simulink model "ES106A_StHlthSigStc"  (R2013b)
settings: Solver=FixedStepDiscrete  SolverMode=SingleTasking  StartTime=0.0  StopTime=1  FixedStep=0.002  RelTol=1e-3
undefined symbols (not defined in the file): APPL10_CNT_U08, BITSPERBYTE_CNT_U08, ENOTOK_CNT_U08, EOK_CNT_U08, LOWRMASKVAL_CNT_U32, NROFCRCAREA_CNT_U08, NVMAVRGPOSN_CNT_U08, NvmGetErrSts1, NVMMAXPOSN_CNT_U08, NVMMINPOSN_CNT_U08, NVMSAMPLECNTRPOSN_CNT_U08, RAMMAXPOSN_CNT_U08, RAMMINPOSN_CNT_U08, RAMRAWPOSN_CNT_U08, SIGCNT_ULS_U08, SigStcPrmInst, STHLTHMAXVAL_CNT_U08, STHLTHOSAPPL_CNT_U16, StHlthTaskRef1, WORDSIZE_CNT_U08
libraries: simulink x43, NxtrNvM x4, NxtrMax x4, NxtrMin x4, FloatToFixd x3, NxtrLim x2
(part 4 of 5)

== system ES106A_StHlthSigStc/StHlthSigStc/GetSigStcHlthData/If Action Subsystem1/GetSigStcHlthData/Subsystem1 ==
  In1 : Inport
  Bitwise Operator1 : simulink/Logic and Bit Operations/Bitwise Operator  logicop=AND  UseBitMask=on  BitMask=bin2dec('1111111100000000')  BitMaskRealWorld=Stored Integer
  Bitwise Operator2 : simulink/Logic and Bit Operations/Bitwise Operator  logicop=AND  UseBitMask=on  BitMask=bin2dec('11111111')  BitMaskRealWorld=Stored Integer
  CopyRight2 : Subsystem  Description=|  mask(Copyright Information){none=on}
      | Copyright info block.                                               
      |                                                                     
      | Place copyright information at the top of every subsystem in design.
      mask prompts: none "No parameters"
      mask help: Place copyright information at the top of every subsystem in design.
      mask Display:
      | NxtrConf = 'Nexteer Confidential';
      | 
      | sys = bdroot; %handle for the current model ("system")
      | first = get_param(sys,'Created');
      | first = first(end-3:end);  %year is last four digits
      | 
      | last = get_param(sys,'LastModifiedDate');
      | if isempty(last)
      |     last = datestr(now,'yyyy');
      | else
      |     last = last(end-3:end);
      | end
      | 
      | if strcmp(first,last)
      |     fprintf('%s -- Copyright %s Nexteer',NxtrConf,first)
      | else
      |     fprintf('%s -- %s%s- %s Nexteer',NxtrConf,char(169),first,last)
      | end
  Data Type Conversion2 : DataTypeConversion  OutDataTypeStr=uint8
  Data Type Conversion3 : DataTypeConversion  OutDataTypeStr=uint8
  Shift Arithmetic2 : ArithShift  BitShiftNumber=8  BitShiftDirection=Right
  Out1 : Outport
  Out2 : Outport  Port=2
  wires:
  Shift Arithmetic2/1 -> Data Type Conversion2/1
  In1/1 -> Bitwise Operator2/1, Bitwise Operator1/1
  Bitwise Operator2/1 -> Data Type Conversion3/1
  Bitwise Operator1/1 -> Shift Arithmetic2/1
  Data Type Conversion2/1 -> Out1/1
  Data Type Conversion3/1 -> Out2/1

== system ES106A_StHlthSigStc/StHlthSigStc/GetSigStcHlthData/If Action Subsystem1/GetSigStcHlthData/Subsystem2 ==
  In1 : Inport
  Bitwise Operator1 : simulink/Logic and Bit Operations/Bitwise Operator  logicop=AND  UseBitMask=on  BitMask=bin2dec('1111111100000000')  BitMaskRealWorld=Stored Integer
  Bitwise Operator2 : simulink/Logic and Bit Operations/Bitwise Operator  logicop=AND  UseBitMask=on  BitMask=bin2dec('11111111')  BitMaskRealWorld=Stored Integer
  CopyRight2 : Subsystem  Description=|  mask(Copyright Information){none=on}
      | Copyright info block.                                               
      |                                                                     
      | Place copyright information at the top of every subsystem in design.
      mask prompts: none "No parameters"
      mask help: Place copyright information at the top of every subsystem in design.
      mask Display:
      | NxtrConf = 'Nexteer Confidential';
      | 
      | sys = bdroot; %handle for the current model ("system")
      | first = get_param(sys,'Created');
      | first = first(end-3:end);  %year is last four digits
      | 
      | last = get_param(sys,'LastModifiedDate');
      | if isempty(last)
      |     last = datestr(now,'yyyy');
      | else
      |     last = last(end-3:end);
      | end
      | 
      | if strcmp(first,last)
      |     fprintf('%s -- Copyright %s Nexteer',NxtrConf,first)
      | else
      |     fprintf('%s -- %s%s- %s Nexteer',NxtrConf,char(169),first,last)
      | end
  Data Type Conversion2 : DataTypeConversion  OutDataTypeStr=uint8
  Data Type Conversion3 : DataTypeConversion  OutDataTypeStr=uint8
  Shift Arithmetic2 : ArithShift  BitShiftNumber=8  BitShiftDirection=Right
  Out1 : Outport
  Out2 : Outport  Port=2
  wires:
  Shift Arithmetic2/1 -> Data Type Conversion2/1
  In1/1 -> Bitwise Operator2/1, Bitwise Operator1/1
  Bitwise Operator2/1 -> Data Type Conversion3/1
  Bitwise Operator1/1 -> Shift Arithmetic2/1
  Data Type Conversion2/1 -> Out1/1
  Data Type Conversion3/1 -> Out2/1

== system ES106A_StHlthSigStc/StHlthSigStc/GetSigStcHlthData/If Action Subsystem1/GetSigStcHlthData/SuspendAllInterrupts ==

== system ES106A_StHlthSigStc/StHlthSigStc/GetSigStcHlthData/If Action Subsystem1/If Action Subsystem/CopyRight2 ==

== system ES106A_StHlthSigStc/StHlthSigStc/StHlthSigStcInit1/Check Applicability/Do Nothing/Subsystem5 ==

== system ES106A_StHlthSigStc/StHlthSigStc/StHlthSigStcInit1/Check Applicability/Set Nvm Invalid/Subsystem5 ==

== system ES106A_StHlthSigStc/StHlthSigStc/StHlthSigStcInit1/For Simulation Purpose/Merger/CopyRight2 ==

== system ES106A_StHlthSigStc/StHlthSigStc/StHlthSigStcInit1/Prepare a buffer for CRC calculation/Iterator/CopyRight2 ==

== system ES106A_StHlthSigStc/StHlthSigStc/StHlthStcPwrDwn/For Iterator Subsystem/If Action Subsystem/ Ignition cycle lasts for less than 1 second. ==
  RamMaxVal : Inport
  RamMinVal : Inport  Port=2
  SigAvrgVal : Inport  Port=3
  SampleCnt : Inport  Port=4
  Action Port : ActionPort  ActionType=else
  CopyRight2 : Subsystem  Description=|  mask(Copyright Information){none=on}
      | Copyright info block.                                               
      |                                                                     
      | Place copyright information at the top of every subsystem in design.
      mask prompts: none "No parameters"
      mask help: Place copyright information at the top of every subsystem in design.
      mask Display:
      | NxtrConf = 'Nexteer Confidential';
      | 
      | sys = bdroot; %handle for the current model ("system")
      | first = get_param(sys,'Created');
      | first = first(end-3:end);  %year is last four digits
      | 
      | last = get_param(sys,'LastModifiedDate');
      | if isempty(last)
      |     last = datestr(now,'yyyy');
      | else
      |     last = last(end-3:end);
      | end
      | 
      | if strcmp(first,last)
      |     fprintf('%s -- Copyright %s Nexteer',NxtrConf,first)
      | else
      |     fprintf('%s -- %s%s- %s Nexteer',NxtrConf,char(169),first,last)
      | end
  NvmMaxVal : Outport
  NvmMinVal : Outport  Port=2
  NvmAvrgVal : Outport  Port=3
  NvmSampleCnt : Outport  Port=4
  wires:
  RamMaxVal/1 -> NvmMaxVal/1
  RamMinVal/1 -> NvmMinVal/1
  SampleCnt/1 -> NvmSampleCnt/1
  SigAvrgVal/1 -> NvmAvrgVal/1

== system ES106A_StHlthSigStc/StHlthSigStc/StHlthStcPwrDwn/For Iterator Subsystem/If Action Subsystem/CopyRight2 ==

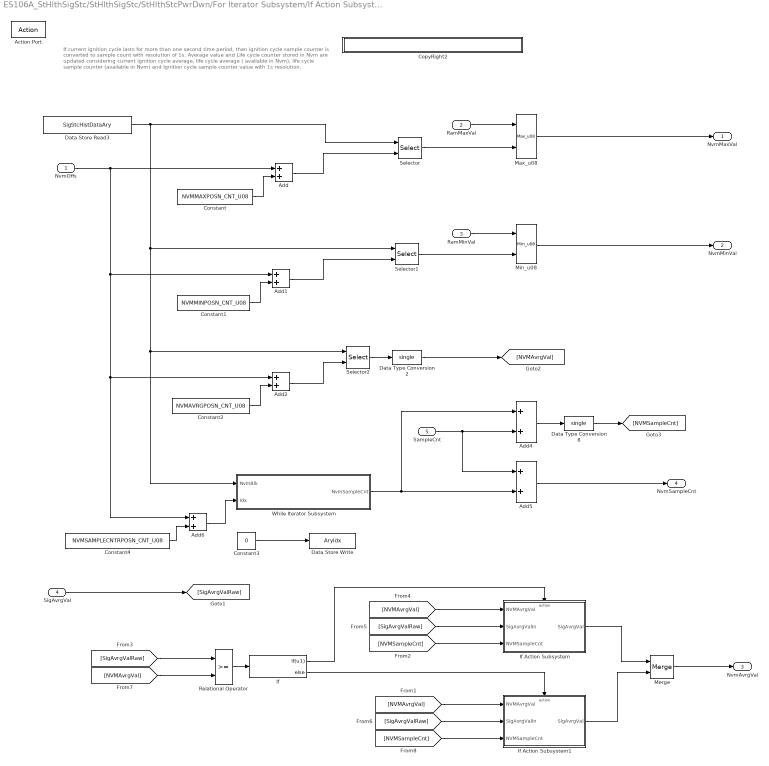
== system ES106A_StHlthSigStc/StHlthSigStc/StHlthStcPwrDwn/For Iterator Subsystem/If Action Subsystem/Statistical data computation for Controller Life Cycle ==
  note: If current ignition cycle lasts for more than one second time period, then ignition cycle sample counter
      | is converted to sample count with resolution of 1s. Average value and Life cycle counter stored in Nvm
      | are updated considering current ignition cycle average, life cycle average ( available in Nvm),
      | life cycle sample counter (available in Nvm) and Ignition cycle sample counter value with 1s resolution.
  NvmOffs : Inport
  RamMaxVal : Inport  Port=2
  RamMinVal : Inport  Port=3
  SigAvrgVal : Inport  Port=4
  SampleCnt : Inport  Port=5
  Action Port : ActionPort  ActionType=then
  Add{,1..2,4..6} (6 alike) : Sum
  Constant : Constant  Value=NVMMAXPOSN_CNT_U08  OutDataTypeStr=uint8
  Constant1 : Constant  Value=NVMMINPOSN_CNT_U08  OutDataTypeStr=uint8
  Constant2 : Constant  Value=NVMAVRGPOSN_CNT_U08  OutDataTypeStr=uint8
  Constant3 : Constant  Value=0
  Constant4 : Constant  Value=NVMSAMPLECNTRPOSN_CNT_U08  OutDataTypeStr=uint8
  CopyRight2 : Subsystem  Description=|  mask(Copyright Information){none=on}
      | Copyright info block.                                               
      |                                                                     
      | Place copyright information at the top of every subsystem in design.
      mask prompts: none "No parameters"
      mask help: Place copyright information at the top of every subsystem in design.
      mask Display:
      | NxtrConf = 'Nexteer Confidential';
      | 
      | sys = bdroot; %handle for the current model ("system")
      | first = get_param(sys,'Created');
      | first = first(end-3:end);  %year is last four digits
      | 
      | last = get_param(sys,'LastModifiedDate');
      | if isempty(last)
      |     last = datestr(now,'yyyy');
      | else
      |     last = last(end-3:end);
      | end
      | 
      | if strcmp(first,last)
      |     fprintf('%s -- Copyright %s Nexteer',NxtrConf,first)
      | else
      |     fprintf('%s -- %s%s- %s Nexteer',NxtrConf,char(169),first,last)
      | end
  Data Store Read3 : DataStoreRead  DataStoreName=SigStcHistDataAry
  Data Store Write : DataStoreWrite  Priority=2  DataStoreName=AryIdx
  Data Type Conversion2 : DataTypeConversion  OutDataTypeStr=single
  Data Type Conversion8 : DataTypeConversion  OutDataTypeStr=single
  If : If  IfExpression=u1
  If Action Subsystem : Subsystem  TreatAsAtomicUnit=on
  If Action Subsystem1 : Subsystem  TreatAsAtomicUnit=on
  Max_u08 : NxtrMax/Max_u08  SFunctionSpec="uint8 y1 = Max_u08( uint8 u1,  uint8 u2)"
      settings: AttributesFormatString=%<Name>
  Merge : Merge
  Min_u08 : NxtrMin/Min_u08  SFunctionSpec="uint8 y1 = Min_u08( uint8 u1,  uint8 u2)"  ShowSpec=off
      settings: AttributesFormatString=%<Name>
  Relational Operator : RelationalOperator  OutDataTypeStr=boolean
  Selector : Selector  IndexMode=Zero-based  InputPortWidth=225  IndexOptions=Starting index (port)  Indices=[1 3]  OutputSizes=1
  Selector1 : Selector  IndexMode=Zero-based  InputPortWidth=225  IndexOptions=Starting index (port)  Indices=[1 3]  OutputSizes=1
  Selector2 : Selector  IndexMode=Zero-based  InputPortWidth=225  IndexOptions=Starting index (port)  Indices=[1 3]  OutputSizes=1
  While Iterator Subsystem : Subsystem  TreatAsAtomicUnit=on
  NvmMaxVal : Outport
  NvmMinVal : Outport  Port=2
  NvmAvrgVal : Outport  Port=3
  NvmSampleCnt : Outport  Port=4
  wires:
  Constant/1 -> Add/2
  Add/1 -> Selector/2
  Constant1/1 -> Add1/2
  Add1/1 -> Selector1/2
  NvmOffs/1 -> Add6/1, Add2/1, Add1/1, Add/1
  Constant2/1 -> Add2/2
  Add2/1 -> Selector2/2
  RamMaxVal/1 -> Max_u08/1
  Selector/1 -> Max_u08/2
  Max_u08/1 -> NvmMaxVal/1
  RamMinVal/1 -> Min_u08/1
  Selector1/1 -> Min_u08/2
  Min_u08/1 -> NvmMinVal/1
  Selector2/1 -> Data Type Conversion2/1
  SampleCnt/1 -> Add5/1, Add4/2
  Add4/1 -> Data Type Conversion8/1
  Add5/1 -> NvmSampleCnt/1
  While Iterator Subsystem/1(NvmSampleCnt) -> Add5/2, Add4/1
  Add6/1 -> While Iterator Subsystem/2(Idx)
  Constant4/1 -> Add6/2
  Constant3/1 -> Data Store Write/1
  Data Store Read3/1 -> Selector2/1, While Iterator Subsystem/1(NvmBlk), Selector1/1, Selector/1
  Relational Operator/1 -> If/1
  If/1 -> If Action Subsystem/Action
  If/2 -> If Action Subsystem1/Action
  Merge/1 -> NvmAvrgVal/1
  If Action Subsystem/1(SigAvrgVal) -> Merge/1
  If Action Subsystem1/1(SigAvrgVal) -> Merge/2
  [NVMAvrgVal] -> If Action Subsystem/1(NVMAvrgVal)
  [NVMAvrgVal] -> If Action Subsystem1/1(NVMAvrgVal)
  [SigAvrgValRaw] -> Relational Operator/1
  Data Type Conversion2/1 -> [NVMAvrgVal]
  [NVMAvrgVal] -> Relational Operator/2
  [NVMSampleCnt] -> If Action Subsystem1/3(NVMSampleCnt)
  [SigAvrgValRaw] -> If Action Subsystem/2(SigAvrgValIn)
  [NVMSampleCnt] -> If Action Subsystem/3(NVMSampleCnt)
  [SigAvrgValRaw] -> If Action Subsystem1/2(SigAvrgValIn)
  SigAvrgVal/1 -> [SigAvrgValRaw]
  Data Type Conversion8/1 -> [NVMSampleCnt]

== system ES106A_StHlthSigStc/StHlthSigStc/StHlthStcPwrDwn/For Iterator Subsystem/If Action Subsystem/Update Nvm ==
  NvmOffset : Inport
  MaxVal : Inport  Port=2
  MinVal : Inport  Port=3
  AvgVal : Inport  Port=4
  SampleCnt : Inport  Port=5
  Assignment : Assignment  IndexMode=Zero-based  IndexOptions=Starting index (port)  Indices=1  OutputSizes=1
  CopyRight2 : Subsystem  Description=|  mask(Copyright Information){none=on}
      | Copyright info block.                                               
      |                                                                     
      | Place copyright information at the top of every subsystem in design.
      mask prompts: none "No parameters"
      mask help: Place copyright information at the top of every subsystem in design.
      mask Display:
      | NxtrConf = 'Nexteer Confidential';
      | 
      | sys = bdroot; %handle for the current model ("system")
      | first = get_param(sys,'Created');
      | first = first(end-3:end);  %year is last four digits
      | 
      | last = get_param(sys,'LastModifiedDate');
      | if isempty(last)
      |     last = datestr(now,'yyyy');
      | else
      |     last = last(end-3:end);
      | end
      | 
      | if strcmp(first,last)
      |     fprintf('%s -- Copyright %s Nexteer',NxtrConf,first)
      | else
      |     fprintf('%s -- %s%s- %s Nexteer',NxtrConf,char(169),first,last)
      | end
  Data Store Read7 : DataStoreRead  DataStoreName=SigStcHistDataAry
  Data Store Write1 : DataStoreWrite  DataStoreName=SigStcHistDataAry
  FloatToFixd_u16_f32 : FloatToFixd/FloatToFixd_u16_f32  Param1=9
  Mux : Mux  Inputs=8
  Subsystem : Subsystem
  Subsystem1 : Subsystem
  wires:
  SampleCnt/1 -> Subsystem/1(In1)
  Assignment/1 -> Data Store Write1/1
  Data Store Read7/1 -> Assignment/1
  Mux/1 -> Assignment/2
  NvmOffset/1 -> Assignment/3
  MaxVal/1 -> Mux/1
  MinVal/1 -> Mux/2
  Subsystem/1(Out1) -> Mux/5
  Subsystem/2(Out2) -> Mux/6
  Subsystem/3(Out3) -> Mux/7
  Subsystem/4(Out4) -> Mux/8
  AvgVal/1 -> FloatToFixd_u16_f32/1
  Subsystem1/1(Out1) -> Mux/3
  Subsystem1/2(Out2) -> Mux/4
  FloatToFixd_u16_f32/1 -> Subsystem1/1(In1)

== system ES106A_StHlthSigStc/StHlthSigStc/UpdStHlthStcData/Call Non Trusted Function /For Iterator Subsystem/CopyRight2 ==

== system ES106A_StHlthSigStc/StHlthSigStc/UpdStHlthStcData/Call Non Trusted Function /For Iterator Subsystem/If Action Subsystem2 ==
  note: /*Do Nothing*/
  Action Port : ActionPort  ActionType=else
  CopyRight2 : Subsystem  Description=|  mask(Copyright Information){none=on}
      | Copyright info block.                                               
      |                                                                     
      | Place copyright information at the top of every subsystem in design.
      mask prompts: none "No parameters"
      mask help: Place copyright information at the top of every subsystem in design.
      mask Display:
      | NxtrConf = 'Nexteer Confidential';
      | 
      | sys = bdroot; %handle for the current model ("system")
      | first = get_param(sys,'Created');
      | first = first(end-3:end);  %year is last four digits
      | 
      | last = get_param(sys,'LastModifiedDate');
      | if isempty(last)
      |     last = datestr(now,'yyyy');
      | else
      |     last = last(end-3:end);
      | end
      | 
      | if strcmp(first,last)
      |     fprintf('%s -- Copyright %s Nexteer',NxtrConf,first)
      | else
      |     fprintf('%s -- %s%s- %s Nexteer',NxtrConf,char(169),first,last)
      | end

== system ES106A_StHlthSigStc/StHlthSigStc/UpdStHlthStcData/Call Non Trusted Function /For Iterator Subsystem/Subsystem2 ==
  note: The Function pointer is terminated in the model to indicate that the pointer
      | points to a location that is outside this FDD. And whiile coding, this pointer is used
      | to access information that is generated from other components.
  FunPtr : Inport
  RAMOffset : Inport  Port=2
  SigIdx : Inport  Port=3
  StHlthSig : Inport  Port=4
  Action Port : ActionPort  ActionType=then
  CopyRight2 : Subsystem  Description=|  mask(Copyright Information){none=on}
      | Copyright info block.                                               
      |                                                                     
      | Place copyright information at the top of every subsystem in design.
      mask prompts: none "No parameters"
      mask help: Place copyright information at the top of every subsystem in design.
      mask Display:
      | NxtrConf = 'Nexteer Confidential';
      | 
      | sys = bdroot; %handle for the current model ("system")
      | first = get_param(sys,'Created');
      | first = first(end-3:end);  %year is last four digits
      | 
      | last = get_param(sys,'LastModifiedDate');
      | if isempty(last)
      |     last = datestr(now,'yyyy');
      | else
      |     last = last(end-3:end);
      | end
      | 
      | if strcmp(first,last)
      |     fprintf('%s -- Copyright %s Nexteer',NxtrConf,first)
      | else
      |     fprintf('%s -- %s%s- %s Nexteer',NxtrConf,char(169),first,last)
      | end
  If Action Subsystem : Subsystem  RequirementInfo={'linktype_rmi_doors' '0001022b (/ESG Group/FDD Module Requirements/EA4 Specific/ES106A_StHlthSigStc )' '#ES106A_15' 'true' 'REQ:ES106A_15' '' ; 'linktype_rmi_doors' '0001022b (/ESG Group/FDD Module Requirements/EA4 Specific/ES106A_StHlthSigStc )' '#ES106A_18' 'true' 'REQ:ES106A_18' '' ; 'linktype_rmi_doors' '0001022b (/ESG Group/FDD Module Requirements/EA4 Specific/ES106A_StHlthSigStc )' '#ES106A_21' 'true' 'REQ:ES106A_21' '' ; 'linktype_rmi_doors' '0001022b (/ESG Group/FDD Module Requirements/EA4 Specific/ES106A_StHlthSigStc )' '#ES106A_22' 'true' 'REQ:ES106A_22' '' } %GIDa_4259b254_6da3_458f_aa6d_9446d195bc64  TreatAsAtomicUnit=on
  Selector : Selector  IndexMode=Zero-based  InputPortWidth=22  IndexOptions=Starting index (port)  Indices=[1 3]  OutputSizes=1
  Terminator : Terminator
  UpdateRamBuf : Subsystem
  UpdateSigAvrgBuf : Subsystem
  wires:
  FunPtr/1 -> Terminator/1
  StHlthSig/1 -> Selector/1
  SigIdx/1 -> [SigIdxVal], Selector/2
  [SigIdxVal] -> If Action Subsystem/1(SigIdx)
  Selector/1 -> If Action Subsystem/2(StHlthSig)
  RAMOffset/1 -> [RAMOffset], If Action Subsystem/3(RAMOffset)
  [RAMOffset] -> UpdateRamBuf/1(RAMLocation)
  If Action Subsystem/1(RamRawVal) -> UpdateRamBuf/2(RamRawVal)
  If Action Subsystem/2(RamMaxVal) -> UpdateRamBuf/3(RamMaxVal)
  If Action Subsystem/3(RamMinVal) -> UpdateRamBuf/4(RamMinVal)
  [SigIdxVal] -> [SigOffset], If Action Subsystem/4(SigOffset)
  [SigOffset] -> UpdateSigAvrgBuf/1(SigAvrgLocation)
  If Action Subsystem/4(SigAvrgVal) -> UpdateSigAvrgBuf/2(SigAvrgVal)

== system ES106A_StHlthSigStc/StHlthSigStc/UpdStHlthStcData/UpdDataSample/For Iterator Subsystem/CopyRight2 ==

== system ES106A_StHlthSigStc/StHlthSigStc/UpdStHlthStcData/UpdDataSample/For Iterator Subsystem/If Action Subsystem2 ==
  note: /*Do Nothing*/
  Action Port : ActionPort  ActionType=else
  CopyRight2 : Subsystem  Description=|  mask(Copyright Information){none=on}
      | Copyright info block.                                               
      |                                                                     
      | Place copyright information at the top of every subsystem in design.
      mask prompts: none "No parameters"
      mask help: Place copyright information at the top of every subsystem in design.
      mask Display:
      | NxtrConf = 'Nexteer Confidential';
      | 
      | sys = bdroot; %handle for the current model ("system")
      | first = get_param(sys,'Created');
      | first = first(end-3:end);  %year is last four digits
      | 
      | last = get_param(sys,'LastModifiedDate');
      | if isempty(last)
      |     last = datestr(now,'yyyy');
      | else
      |     last = last(end-3:end);
      | end
      | 
      | if strcmp(first,last)
      |     fprintf('%s -- Copyright %s Nexteer',NxtrConf,first)
      | else
      |     fprintf('%s -- %s%s- %s Nexteer',NxtrConf,char(169),first,last)
      | end

== system ES106A_StHlthSigStc/StHlthSigStc/UpdStHlthStcData/UpdDataSample/For Iterator Subsystem/Subsystem2 ==
  note: The Function pointer is terminated in the model to indicate that the pointer
      | points to a location that is outside this FDD. And whiile coding, this pointer is used
      | to access information that is generated from other components.
  FunPtr : Inport
  RAMOffset : Inport  Port=2
  SigIdx : Inport  Port=3
  StHlthSig : Inport  Port=4
  Action Port : ActionPort  ActionType=then
  CopyRight2 : Subsystem  Description=|  mask(Copyright Information){none=on}
      | Copyright info block.                                               
      |                                                                     
      | Place copyright information at the top of every subsystem in design.
      mask prompts: none "No parameters"
      mask help: Place copyright information at the top of every subsystem in design.
      mask Display:
      | NxtrConf = 'Nexteer Confidential';
      | 
      | sys = bdroot; %handle for the current model ("system")
      | first = get_param(sys,'Created');
      | first = first(end-3:end);  %year is last four digits
      | 
      | last = get_param(sys,'LastModifiedDate');
      | if isempty(last)
      |     last = datestr(now,'yyyy');
      | else
      |     last = last(end-3:end);
      | end
      | 
      | if strcmp(first,last)
      |     fprintf('%s -- Copyright %s Nexteer',NxtrConf,first)
      | else
      |     fprintf('%s -- %s%s- %s Nexteer',NxtrConf,char(169),first,last)
      | end
  If Action Subsystem : Subsystem  RequirementInfo={'linktype_rmi_doors' '0001022b (/ESG Group/FDD Module Requirements/EA4 Specific/ES106A_StHlthSigStc )' '#ES106A_15' 'true' 'REQ:ES106A_15' '' ; 'linktype_rmi_doors' '0001022b (/ESG Group/FDD Module Requirements/EA4 Specific/ES106A_StHlthSigStc )' '#ES106A_18' 'true' 'REQ:ES106A_18' '' ; 'linktype_rmi_doors' '0001022b (/ESG Group/FDD Module Requirements/EA4 Specific/ES106A_StHlthSigStc )' '#ES106A_21' 'true' 'REQ:ES106A_21' '' ; 'linktype_rmi_doors' '0001022b (/ESG Group/FDD Module Requirements/EA4 Specific/ES106A_StHlthSigStc )' '#ES106A_22' 'true' 'REQ:ES106A_22' '' } %GIDa_dda2dc3d_9a01_4c14_a4da_d10ab0df32b8  TreatAsAtomicUnit=on
  Selector : Selector  IndexMode=Zero-based  InputPortWidth=22  IndexOptions=Starting index (port)  Indices=[1 3]  OutputSizes=1
  Terminator : Terminator
  UpdateRamBuf : Subsystem
  UpdateSigAvrgBuf : Subsystem
  wires:
  FunPtr/1 -> Terminator/1
  StHlthSig/1 -> Selector/1
  SigIdx/1 -> [SigIdxVal], Selector/2
  [SigIdxVal] -> If Action Subsystem/1(SigIdx)
  Selector/1 -> If Action Subsystem/2(StHlthSig)
  RAMOffset/1 -> [RAMOffset], If Action Subsystem/3(RAMOffset)
  [RAMOffset] -> UpdateRamBuf/1(RAMLocation)
  If Action Subsystem/1(RamRawVal) -> UpdateRamBuf/2(RamRawVal)
  If Action Subsystem/2(RamMaxVal) -> UpdateRamBuf/3(RamMaxVal)
  If Action Subsystem/3(RamMinVal) -> UpdateRamBuf/4(RamMinVal)
  [SigIdxVal] -> [SigOffset], If Action Subsystem/4(SigAvrgOffset)
  [SigOffset] -> UpdateSigAvrgBuf/1(SigAvrgLocation)
  If Action Subsystem/4(SigAvrgVal) -> UpdateSigAvrgBuf/2(SigAvrgVal)

== system ES106A_StHlthSigStc/StHlthSigStc/GetSigStcHlthData/If Action Subsystem1/GetSigStcHlthData/If Action Subsystem/CopyRight2 ==

== system ES106A_StHlthSigStc/StHlthSigStc/GetSigStcHlthData/If Action Subsystem1/GetSigStcHlthData/If Action Subsystem/If Action Subsystem ==
  NVMAvrgVal : Inport
  SigAvrgValIn : Inport  Port=2
  NVMSampleCnt : Inport  Port=3
  Action Port : ActionPort  ActionType=then
  Add1 : Sum
  Add4 : Sum  Inputs=+-
  Divide : Product  Inputs=*/
  SigAvrgVal : Outport
  wires:
  [SigAvrgVal] -> Add4/1
  NVMAvrgVal/1 -> [NVMAvrgVal]
  Add4/1 -> Divide/1
  NVMSampleCnt/1 -> Divide/2
  SigAvrgValIn/1 -> [SigAvrgVal]
  Divide/1 -> Add1/2
  [NVMAvrgVal] -> Add1/1
  Add1/1 -> SigAvrgVal/1
  [NVMAvrgVal] -> Add4/2

== system ES106A_StHlthSigStc/StHlthSigStc/GetSigStcHlthData/If Action Subsystem1/GetSigStcHlthData/If Action Subsystem/If Action Subsystem1 ==
  NVMAvrgVal : Inport
  SigAvrgValIn : Inport  Port=2
  NVMSampleCnt : Inport  Port=3
  Action Port : ActionPort  ActionType=else
  Add1 : Sum  Inputs=+-
  Add4 : Sum  Inputs=+-
  Divide : Product  Inputs=*/
  SigAvrgVal : Outport
  wires:
  [SigAvrgVal] -> Add4/2
  NVMAvrgVal/1 -> [NVMAvrgVal]
  Add4/1 -> Divide/1
  NVMSampleCnt/1 -> Divide/2
  SigAvrgValIn/1 -> [SigAvrgVal]
  Divide/1 -> Add1/2
  [NVMAvrgVal] -> Add1/1
  Add1/1 -> SigAvrgVal/1
  [NVMAvrgVal] -> Add4/1

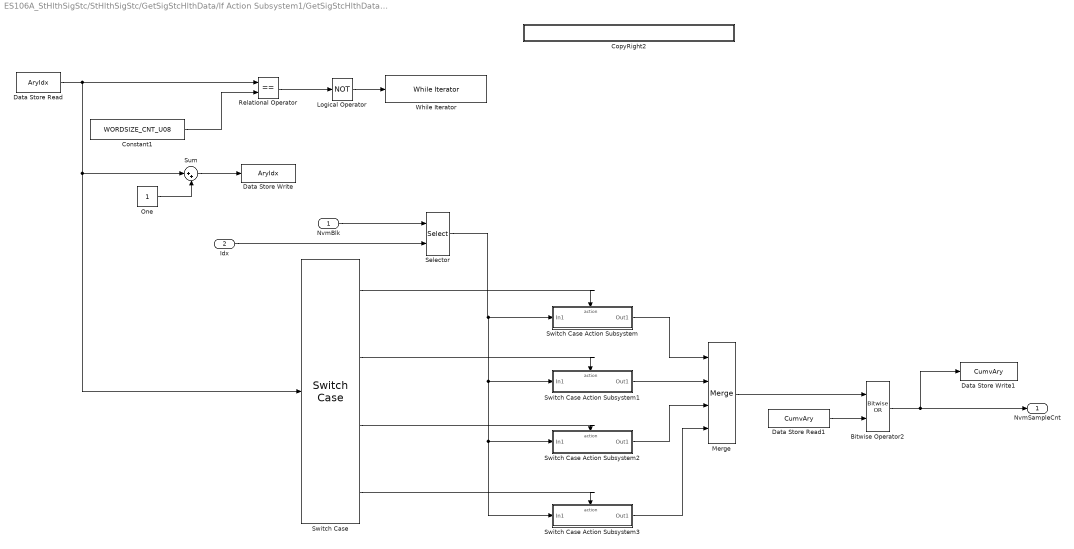
== system ES106A_StHlthSigStc/StHlthSigStc/GetSigStcHlthData/If Action Subsystem1/GetSigStcHlthData/If Action Subsystem/While Iterator Subsystem ==
  NvmBlk : Inport
  Idx : Inport  Port=2
  Bitwise Operator2 : simulink/Logic and Bit Operations/Bitwise Operator  logicop=OR  UseBitMask=off  NumInputPorts=2  BitMask=bin2dec('11011001')  BitMaskRealWorld=Stored Integer
  Constant1 : Constant  Value=WORDSIZE_CNT_U08
  CopyRight2 : Subsystem  Description=|  mask(Copyright Information){none=on}
      | Copyright info block.                                               
      |                                                                     
      | Place copyright information at the top of every subsystem in design.
      mask prompts: none "No parameters"
      mask help: Place copyright information at the top of every subsystem in design.
      mask Display:
      | NxtrConf = 'Nexteer Confidential';
      | 
      | sys = bdroot; %handle for the current model ("system")
      | first = get_param(sys,'Created');
      | if(isempty(first))
      |     first = datestr(now,'yyyy');
      | else
      |     first = first(end-3:end);  %year is last four digits
      | end
      | 
      | last = get_param(sys,'LastModifiedDate');
      | if isempty(last)
      |     last = datestr(now,'yyyy');
      | else
      |     last = last(end-3:end);
      | end
      | 
      | if strcmp(first,last)
      |     fprintf('%s -- Copyright %s Nexteer',NxtrConf,first)
      | else
      |     fprintf('%s -- %s%s- %s Nexteer',NxtrConf,char(169),first,last)
      | end
  Data Store Read : DataStoreRead  Priority=1  DataStoreName=AryIdx
      settings: AttributesFormatString=PRIORITY: %<Priority>
  Data Store Read1 : DataStoreRead  Priority=1  DataStoreName=CumvAry
      settings: AttributesFormatString=Priority:%<Priority>
  Data Store Write : DataStoreWrite  Priority=2  DataStoreName=AryIdx
      settings: AttributesFormatString=PRIORITY:%<Priority>
  Data Store Write1 : DataStoreWrite  Priority=2  DataStoreName=CumvAry
      settings: AttributesFormatString=Priority:%<Priority>
  Logical Operator : Logic  Operator=NOT  AllPortsSameDT=off  OutDataTypeStr=boolean
  Merge : Merge  Inputs=4
  One : Constant
  Relational Operator : RelationalOperator  Operator===  OutDataTypeStr=boolean
  Selector : Selector  IndexMode=Zero-based  InputPortWidth=225  IndexOptions=Index vector (port)  Indices=[1 3]  OutputSizes=1
  Sum : Sum  Inputs=|++
  Switch Case : SwitchCase  CaseConditions={0,1,2,3}  ShowDefaultCase=off
  Switch Case Action Subsystem : Subsystem  TreatAsAtomicUnit=on
  Switch Case Action Subsystem1 : Subsystem  TreatAsAtomicUnit=on
  Switch Case Action Subsystem2 : Subsystem  TreatAsAtomicUnit=on
  Switch Case Action Subsystem3 : Subsystem  TreatAsAtomicUnit=on
  While Iterator : WhileIterator  WhileBlockType=do-while
  NvmSampleCnt : Outport
  wires:
  Relational Operator/1 -> Logical Operator/1
  One/1 -> Sum/2
  Sum/1 -> Data Store Write/1
  NvmBlk/1 -> Selector/1
  Bitwise Operator2/1 -> NvmSampleCnt/1, Data Store Write1/1
  Selector/1 -> Switch Case Action Subsystem3/1(In1), Switch Case Action Subsystem2/1(In1), Switch Case Action Subsystem1/1(In1), Switch Case Action Subsystem/1(In1)
  Data Store Read1/1 -> Bitwise Operator2/2
  Data Store Read/1 -> Relational Operator/1, Sum/1, Switch Case/1
  Switch Case/1 -> Switch Case Action Subsystem/Action
  Switch Case/2 -> Switch Case Action Subsystem1/Action
  Switch Case/3 -> Switch Case Action Subsystem2/Action
  Switch Case/4 -> Switch Case Action Subsystem3/Action
  Switch Case Action Subsystem/1(Out1) -> Merge/1
  Switch Case Action Subsystem1/1(Out1) -> Merge/2
  Switch Case Action Subsystem2/1(Out1) -> Merge/3
  Switch Case Action Subsystem3/1(Out1) -> Merge/4
  Merge/1 -> Bitwise Operator2/1
  Logical Operator/1 -> While Iterator/1
  Constant1/1 -> Relational Operator/2
  Idx/1 -> Selector/2

== system ES106A_StHlthSigStc/StHlthSigStc/GetSigStcHlthData/If Action Subsystem1/GetSigStcHlthData/If Action Subsystem1/CopyRight2 ==

== system ES106A_StHlthSigStc/StHlthSigStc/GetSigStcHlthData/If Action Subsystem1/GetSigStcHlthData/Subsystem/CopyRight2 ==

== system ES106A_StHlthSigStc/StHlthSigStc/GetSigStcHlthData/If Action Subsystem1/GetSigStcHlthData/Subsystem1/CopyRight2 ==

== system ES106A_StHlthSigStc/StHlthSigStc/GetSigStcHlthData/If Action Subsystem1/GetSigStcHlthData/Subsystem2/CopyRight2 ==

== system ES106A_StHlthSigStc/StHlthSigStc/StHlthStcPwrDwn/For Iterator Subsystem/If Action Subsystem/ Ignition cycle lasts for less than 1 second./CopyRight2 ==

== system ES106A_StHlthSigStc/StHlthSigStc/StHlthStcPwrDwn/For Iterator Subsystem/If Action Subsystem/Statistical data computation for Controller Life Cycle/CopyRight2 ==

== system ES106A_StHlthSigStc/StHlthSigStc/StHlthStcPwrDwn/For Iterator Subsystem/If Action Subsystem/Statistical data computation for Controller Life Cycle/If Action Subsystem ==
  NVMAvrgVal : Inport
  SigAvrgValIn : Inport  Port=2
  NVMSampleCnt : Inport  Port=3
  Action Port : ActionPort  ActionType=then
  Add1 : Sum
  Add4 : Sum  Inputs=+-
  Divide : Product  Inputs=*/
  SigAvrgVal : Outport
  wires:
  [SigAvrgVal] -> Add4/1
  NVMAvrgVal/1 -> [NVMAvrgVal]
  Add4/1 -> Divide/1
  NVMSampleCnt/1 -> Divide/2
  SigAvrgValIn/1 -> [SigAvrgVal]
  Divide/1 -> Add1/2
  [NVMAvrgVal] -> Add1/1
  Add1/1 -> SigAvrgVal/1
  [NVMAvrgVal] -> Add4/2

== system ES106A_StHlthSigStc/StHlthSigStc/StHlthStcPwrDwn/For Iterator Subsystem/If Action Subsystem/Statistical data computation for Controller Life Cycle/If Action Subsystem1 ==
  NVMAvrgVal : Inport
  SigAvrgValIn : Inport  Port=2
  NVMSampleCnt : Inport  Port=3
  Action Port : ActionPort  ActionType=else
  Add1 : Sum  Inputs=+-
  Add4 : Sum  Inputs=+-
  Divide : Product  Inputs=*/
  SigAvrgVal : Outport
  wires:
  [SigAvrgVal] -> Add4/2
  NVMAvrgVal/1 -> [NVMAvrgVal]
  Add4/1 -> Divide/1
  NVMSampleCnt/1 -> Divide/2
  SigAvrgValIn/1 -> [SigAvrgVal]
  Divide/1 -> Add1/2
  [NVMAvrgVal] -> Add1/1
  Add1/1 -> SigAvrgVal/1
  [NVMAvrgVal] -> Add4/1

== system ES106A_StHlthSigStc/StHlthSigStc/StHlthStcPwrDwn/For Iterator Subsystem/If Action Subsystem/Statistical data computation for Controller Life Cycle/While Iterator Subsystem ==
  NvmBlk : Inport
  Idx : Inport  Port=2
  Bitwise Operator2 : simulink/Logic and Bit Operations/Bitwise Operator  logicop=OR  UseBitMask=off  NumInputPorts=2  BitMask=bin2dec('11011001')  BitMaskRealWorld=Stored Integer
  Constant1 : Constant  Value=WORDSIZE_CNT_U08
  CopyRight2 : Subsystem  Description=|  mask(Copyright Information){none=on}
      | Copyright info block.                                               
      |                                                                     
      | Place copyright information at the top of every subsystem in design.
      mask prompts: none "No parameters"
      mask help: Place copyright information at the top of every subsystem in design.
      mask Display:
      | NxtrConf = 'Nexteer Confidential';
      | 
      | sys = bdroot; %handle for the current model ("system")
      | first = get_param(sys,'Created');
      | if(isempty(first))
      |     first = datestr(now,'yyyy');
      | else
      |     first = first(end-3:end);  %year is last four digits
      | end
      | 
      | last = get_param(sys,'LastModifiedDate');
      | if isempty(last)
      |     last = datestr(now,'yyyy');
      | else
      |     last = last(end-3:end);
      | end
      | 
      | if strcmp(first,last)
      |     fprintf('%s -- Copyright %s Nexteer',NxtrConf,first)
      | else
      |     fprintf('%s -- %s%s- %s Nexteer',NxtrConf,char(169),first,last)
      | end
  Data Store Read : DataStoreRead  Priority=1  DataStoreName=AryIdx
      settings: AttributesFormatString=PRIORITY: %<Priority>
  Data Store Read1 : DataStoreRead  Priority=1  DataStoreName=CumvAry
      settings: AttributesFormatString=Priority:%<Priority>
  Data Store Write : DataStoreWrite  Priority=2  DataStoreName=AryIdx
      settings: AttributesFormatString=PRIORITY:%<Priority>
  Data Store Write1 : DataStoreWrite  Priority=2  DataStoreName=CumvAry
      settings: AttributesFormatString=Priority:%<Priority>
  Logical Operator : Logic  Operator=NOT  AllPortsSameDT=off  OutDataTypeStr=boolean
  Merge : Merge  Inputs=4
  One : Constant
  Relational Operator : RelationalOperator  Operator===  OutDataTypeStr=boolean
  Selector : Selector  IndexMode=Zero-based  InputPortWidth=225  IndexOptions=Index vector (port)  Indices=[1 3]  OutputSizes=1
  Sum : Sum  Inputs=|++
  Switch Case : SwitchCase  CaseConditions={0,1,2,3}  ShowDefaultCase=off
  Switch Case Action Subsystem : Subsystem  TreatAsAtomicUnit=on
  Switch Case Action Subsystem1 : Subsystem  TreatAsAtomicUnit=on
  Switch Case Action Subsystem2 : Subsystem  TreatAsAtomicUnit=on
  Switch Case Action Subsystem3 : Subsystem  TreatAsAtomicUnit=on
  While Iterator : WhileIterator  WhileBlockType=do-while
  NvmSampleCnt : Outport
  wires:
  Relational Operator/1 -> Logical Operator/1
  One/1 -> Sum/2
  Sum/1 -> Data Store Write/1
  NvmBlk/1 -> Selector/1
  Bitwise Operator2/1 -> NvmSampleCnt/1, Data Store Write1/1
  Selector/1 -> Switch Case Action Subsystem3/1(In1), Switch Case Action Subsystem2/1(In1), Switch Case Action Subsystem1/1(In1), Switch Case Action Subsystem/1(In1)
  Data Store Read1/1 -> Bitwise Operator2/2
  Data Store Read/1 -> Relational Operator/1, Sum/1, Switch Case/1
  Switch Case/1 -> Switch Case Action Subsystem/Action
  Switch Case/2 -> Switch Case Action Subsystem1/Action
  Switch Case/3 -> Switch Case Action Subsystem2/Action
  Switch Case/4 -> Switch Case Action Subsystem3/Action
  Switch Case Action Subsystem/1(Out1) -> Merge/1
  Switch Case Action Subsystem1/1(Out1) -> Merge/2
  Switch Case Action Subsystem2/1(Out1) -> Merge/3
  Switch Case Action Subsystem3/1(Out1) -> Merge/4
  Merge/1 -> Bitwise Operator2/1
  Logical Operator/1 -> While Iterator/1
  Constant1/1 -> Relational Operator/2
  Idx/1 -> Selector/2

== system ES106A_StHlthSigStc/StHlthSigStc/StHlthStcPwrDwn/For Iterator Subsystem/If Action Subsystem/Update Nvm/CopyRight2 ==

== system ES106A_StHlthSigStc/StHlthSigStc/StHlthStcPwrDwn/For Iterator Subsystem/If Action Subsystem/Update Nvm/Subsystem ==
  In1 : Inport  OutDataTypeStr=uint32
  Bitwise Operator : simulink/Logic and Bit Operations/Bitwise Operator  logicop=AND  UseBitMask=on  BitMask=bin2dec('111111110000000000000000')  BitMaskRealWorld=Stored Integer
  Bitwise Operator1 : simulink/Logic and Bit Operations/Bitwise Operator  logicop=AND  UseBitMask=on  BitMask=bin2dec('1111111100000000')  BitMaskRealWorld=Stored Integer
  Bitwise Operator2 : simulink/Logic and Bit Operations/Bitwise Operator  logicop=AND  UseBitMask=on  BitMask=bin2dec('11111111')  BitMaskRealWorld=Stored Integer
  CopyRight2 : Subsystem  Description=|  mask(Copyright Information){none=on}
      | Copyright info block.                                               
      |                                                                     
      | Place copyright information at the top of every subsystem in design.
      mask prompts: none "No parameters"
      mask help: Place copyright information at the top of every subsystem in design.
      mask Display:
      | NxtrConf = 'Nexteer Confidential';
      | 
      | sys = bdroot; %handle for the current model ("system")
      | first = get_param(sys,'Created');
      | first = first(end-3:end);  %year is last four digits
      | 
      | last = get_param(sys,'LastModifiedDate');
      | if isempty(last)
      |     last = datestr(now,'yyyy');
      | else
      |     last = last(end-3:end);
      | end
      | 
      | if strcmp(first,last)
      |     fprintf('%s -- Copyright %s Nexteer',NxtrConf,first)
      | else
      |     fprintf('%s -- %s%s- %s Nexteer',NxtrConf,char(169),first,last)
      | end
  Data Type Conversion{,1..3} (4 alike) : DataTypeConversion  OutDataTypeStr=uint8
  Shift Arithmetic : ArithShift  BitShiftNumber=16  BitShiftDirection=Right
  Shift Arithmetic1 : ArithShift  BitShiftNumber=24  BitShiftDirection=Right
  Shift Arithmetic2 : ArithShift  BitShiftNumber=8  BitShiftDirection=Right
  Out1 : Outport
  Out2 : Outport  Port=2
  Out3 : Outport  Port=3
  Out4 : Outport  Port=4
  wires:
  Shift Arithmetic2/1 -> Data Type Conversion2/1
  In1/1 -> Shift Arithmetic1/1, Bitwise Operator/1, Bitwise Operator2/1, Bitwise Operator1/1
  Bitwise Operator2/1 -> Data Type Conversion3/1
  Bitwise Operator/1 -> Shift Arithmetic/1
  Shift Arithmetic/1 -> Data Type Conversion1/1
  Shift Arithmetic1/1 -> Data Type Conversion/1
  Bitwise Operator1/1 -> Shift Arithmetic2/1
  Data Type Conversion/1 -> Out1/1
  Data Type Conversion1/1 -> Out2/1
  Data Type Conversion2/1 -> Out3/1
  Data Type Conversion3/1 -> Out4/1

== system ES106A_StHlthSigStc/StHlthSigStc/StHlthStcPwrDwn/For Iterator Subsystem/If Action Subsystem/Update Nvm/Subsystem1 ==
  In1 : Inport
  Bitwise Operator1 : simulink/Logic and Bit Operations/Bitwise Operator  logicop=AND  UseBitMask=on  BitMask=bin2dec('1111111100000000')  BitMaskRealWorld=Stored Integer
  Bitwise Operator2 : simulink/Logic and Bit Operations/Bitwise Operator  logicop=AND  UseBitMask=on  BitMask=bin2dec('11111111')  BitMaskRealWorld=Stored Integer
  CopyRight2 : Subsystem  Description=|  mask(Copyright Information){none=on}
      | Copyright info block.                                               
      |                                                                     
      | Place copyright information at the top of every subsystem in design.
      mask prompts: none "No parameters"
      mask help: Place copyright information at the top of every subsystem in design.
      mask Display:
      | NxtrConf = 'Nexteer Confidential';
      | 
      | sys = bdroot; %handle for the current model ("system")
      | first = get_param(sys,'Created');
      | first = first(end-3:end);  %year is last four digits
      | 
      | last = get_param(sys,'LastModifiedDate');
      | if isempty(last)
      |     last = datestr(now,'yyyy');
      | else
      |     last = last(end-3:end);
      | end
      | 
      | if strcmp(first,last)
      |     fprintf('%s -- Copyright %s Nexteer',NxtrConf,first)
      | else
      |     fprintf('%s -- %s%s- %s Nexteer',NxtrConf,char(169),first,last)
      | end
  Data Type Conversion2 : DataTypeConversion  OutDataTypeStr=uint8
  Data Type Conversion3 : DataTypeConversion  OutDataTypeStr=uint8
  Shift Arithmetic2 : ArithShift  BitShiftNumber=8  BitShiftDirection=Right
  Out1 : Outport
  Out2 : Outport  Port=2
  wires:
  Shift Arithmetic2/1 -> Data Type Conversion2/1
  In1/1 -> Bitwise Operator2/1, Bitwise Operator1/1
  Bitwise Operator2/1 -> Data Type Conversion3/1
  Bitwise Operator1/1 -> Shift Arithmetic2/1
  Data Type Conversion2/1 -> Out1/1
  Data Type Conversion3/1 -> Out2/1

== system ES106A_StHlthSigStc/StHlthSigStc/UpdStHlthStcData/Call Non Trusted Function /For Iterator Subsystem/If Action Subsystem2/CopyRight2 ==

== system ES106A_StHlthSigStc/StHlthSigStc/UpdStHlthStcData/Call Non Trusted Function /For Iterator Subsystem/Subsystem2/CopyRight2 ==

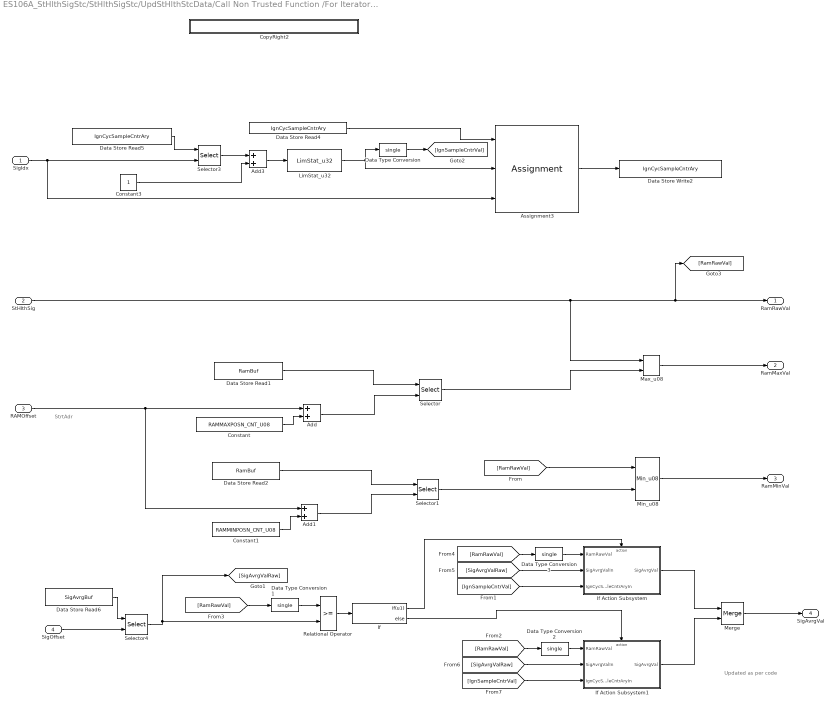
== system ES106A_StHlthSigStc/StHlthSigStc/UpdStHlthStcData/Call Non Trusted Function /For Iterator Subsystem/Subsystem2/If Action Subsystem ==
  note: StrtAdr
  note: Updated as per code
  SigIdx : Inport
  StHlthSig : Inport  Port=2
  RAMOffset : Inport  Port=3
  SigOffset : Inport  Port=4
  Add : Sum
  Add1 : Sum
  Add3 : Sum
  Assignment3 : Assignment  IndexMode=Zero-based  IndexOptions=Starting index (port)  Indices=1  OutputSizes=1
  Constant : Constant  Value=RAMMAXPOSN_CNT_U08  OutDataTypeStr=uint8
      settings: AttributesFormatString=%<OutDataTypeStr>
  Constant1 : Constant  Value=RAMMINPOSN_CNT_U08  OutDataTypeStr=uint8
      settings: AttributesFormatString=%<OutDataTypeStr>
  Constant3 : Constant  OutDataTypeStr=uint8
      settings: AttributesFormatString=%<OutDataTypeStr>
  CopyRight2 : Subsystem  Description=|  mask(Copyright Information){none=on}
      | Copyright info block.                                               
      |                                                                     
      | Place copyright information at the top of every subsystem in design.
      mask prompts: none "No parameters"
      mask help: Place copyright information at the top of every subsystem in design.
      mask Display:
      | NxtrConf = 'Nexteer Confidential';
      | 
      | sys = bdroot; %handle for the current model ("system")
      | first = get_param(sys,'Created');
      | first = first(end-3:end);  %year is last four digits
      | 
      | last = get_param(sys,'LastModifiedDate');
      | if isempty(last)
      |     last = datestr(now,'yyyy');
      | else
      |     last = last(end-3:end);
      | end
      | 
      | if strcmp(first,last)
      |     fprintf('%s -- Copyright %s Nexteer',NxtrConf,first)
      | else
      |     fprintf('%s -- %s%s- %s Nexteer',NxtrConf,char(169),first,last)
      | end
  Data Store Read1 : DataStoreRead  DataStoreName=RamBuf
  Data Store Read2 : DataStoreRead  DataStoreName=RamBuf
  Data Store Read4 : DataStoreRead  Priority=2  DataStoreName=IgnCycSampleCntrAry
      settings: AttributesFormatString=Priority: %<Priority>
  Data Store Read5 : DataStoreRead  Priority=1  DataStoreName=IgnCycSampleCntrAry
      settings: AttributesFormatString=Priority: %<Priority>
  Data Store Read6 : DataStoreRead  DataStoreName=SigAvrgBuf
  Data Store Write2 : DataStoreWrite  Priority=3  DataStoreName=IgnCycSampleCntrAry
      settings: AttributesFormatString=Priority: %<Priority>
  Data Type Conversion{,1..3} (4 alike) : DataTypeConversion  OutDataTypeStr=single
  If : If  IfExpression=u1
  If Action Subsystem : Subsystem  TreatAsAtomicUnit=on
  If Action Subsystem1 : Subsystem  TreatAsAtomicUnit=on
  LimStat_u32 : NxtrLim/LimStat_u32  LoLim=IGNCYCSAMPLECNTRARYMINLIM_CNT_U32  HiLim=IGNCYCSAMPLECNTRARYMAXLIM_CNT_U32
      settings: AttributesFormatString=|
      | Low Limit: %<LoLim>
      | High Limit:%<HiLim>
  Max_u08 : NxtrMax/Max_u08  SFunctionSpec="uint8 y1 = Max_u08( uint8 u1,  uint8 u2)"
      settings: AttributesFormatString=%<Name>
  Merge : Merge
  Min_u08 : NxtrMin/Min_u08  SFunctionSpec="uint8 y1 = Min_u08( uint8 u1,  uint8 u2)"  ShowSpec=off
      settings: AttributesFormatString=%<Name>
  Relational Operator : RelationalOperator  OutDataTypeStr=boolean
  Selector : Selector  IndexMode=Zero-based  InputPortWidth=66  IndexOptions=Starting index (port)  Indices=[1 3]  OutputSizes=1
  Selector1 : Selector  IndexMode=Zero-based  InputPortWidth=66  IndexOptions=Starting index (port)  Indices=[1 3]  OutputSizes=1
  Selector3 : Selector  IndexMode=Zero-based  InputPortWidth=22  IndexOptions=Starting index (port)  Indices=[1 3]  OutputSizes=1
  Selector4 : Selector  IndexMode=Zero-based  InputPortWidth=22  IndexOptions=Starting index (port)  Indices=[1 3]  OutputSizes=1
  RamRawVal : Outport
  RamMaxVal : Outport  Port=2
  RamMinVal : Outport  Port=3
  SigAvrgVal : Outport  Port=4
  wires:
  Data Store Read1/1 -> Selector/1
  Constant/1 -> Add/2
  Add/1 -> Selector/2
  Selector/1 -> Max_u08/2
  Data Store Read2/1 -> Selector1/1
  Constant1/1 -> Add1/2
  Add1/1 -> Selector1/2
  Selector1/1 -> Min_u08/2
  StHlthSig/1 -> [RamRawVal], RamRawVal/1, Max_u08/1
  RAMOffset/1 -> Add1/1, Add/1
  Max_u08/1 -> RamMaxVal/1
  [RamRawVal] -> Min_u08/1
  Min_u08/1 -> RamMinVal/1
  Data Store Read6/1 -> Selector4/1
  Relational Operator/1 -> If/1
  [RamRawVal] -> Data Type Conversion1/1
  If/1 -> If Action Subsystem/Action
  If/2 -> If Action Subsystem1/Action
  Merge/1 -> SigAvrgVal/1
  If Action Subsystem/1(SigAvrgVal) -> Merge/1
  If Action Subsystem1/1(SigAvrgVal) -> Merge/2
  [RamRawVal] -> Data Type Conversion3/1
  [IgnSampleCntrVal] -> If Action Subsystem/3(IgnCycSampleCntrAryIn)
  [RamRawVal] -> Data Type Conversion2/1
  SigOffset/1 -> Selector4/2
  [SigAvrgValRaw] -> If Action Subsystem1/2(SigAvrgValIn)
  [SigAvrgValRaw] -> If Action Subsystem/2(SigAvrgValIn)
  Selector4/1 -> [SigAvrgValRaw], Relational Operator/2
  Data Type Conversion2/1 -> If Action Subsystem1/1(RamRawVal)
  Data Type Conversion3/1 -> If Action Subsystem/1(RamRawVal)
  Data Type Conversion1/1 -> Relational Operator/1
  Data Store Read5/1 -> Selector3/1
  Selector3/1 -> Add3/1
  Constant3/1 -> Add3/2
  Assignment3/1 -> Data Store Write2/1
  Add3/1 -> LimStat_u32/1
  Data Store Read4/1 -> Assignment3/1
  SigIdx/1 -> Assignment3/3, Selector3/2
  LimStat_u32/1 -> Data Type Conversion/1, Assignment3/2
  Data Type Conversion/1 -> [IgnSampleCntrVal]
  [IgnSampleCntrVal] -> If Action Subsystem1/3(IgnCycSampleCntrAryIn)

== system ES106A_StHlthSigStc/StHlthSigStc/UpdStHlthStcData/Call Non Trusted Function /For Iterator Subsystem/Subsystem2/UpdateRamBuf ==
  note: RamAvrgVal signal has been deleted
  RAMLocation : Inport
  RamRawVal : Inport  Port=2
  RamMaxVal : Inport  Port=3
  RamMinVal : Inport  Port=4
  Assignment4 : Assignment  IndexMode=Zero-based  IndexOptions=Starting index (port)  Indices=1  OutputSizes=1
  CopyRight2 : Subsystem  Description=|  mask(Copyright Information){none=on}
      | Copyright info block.                                               
      |                                                                     
      | Place copyright information at the top of every subsystem in design.
      mask prompts: none "No parameters"
      mask help: Place copyright information at the top of every subsystem in design.
      mask Display:
      | NxtrConf = 'Nexteer Confidential';
      | 
      | sys = bdroot; %handle for the current model ("system")
      | first = get_param(sys,'Created');
      | first = first(end-3:end);  %year is last four digits
      | 
      | last = get_param(sys,'LastModifiedDate');
      | if isempty(last)
      |     last = datestr(now,'yyyy');
      | else
      |     last = last(end-3:end);
      | end
      | 
      | if strcmp(first,last)
      |     fprintf('%s -- Copyright %s Nexteer',NxtrConf,first)
      | else
      |     fprintf('%s -- %s%s- %s Nexteer',NxtrConf,char(169),first,last)
      | end
  Data Store Read1 : DataStoreRead  DataStoreName=RamBuf
  Data Store Write2 : DataStoreWrite  DataStoreName=RamBuf
  Mux : Mux  Inputs=3
  wires:
  Data Store Read1/1 -> Assignment4/1
  RAMLocation/1 -> Assignment4/3
  Mux/1 -> Assignment4/2
  Assignment4/1 -> Data Store Write2/1
  RamRawVal/1 -> Mux/1
  RamMaxVal/1 -> Mux/2
  RamMinVal/1 -> Mux/3

== system ES106A_StHlthSigStc/StHlthSigStc/UpdStHlthStcData/Call Non Trusted Function /For Iterator Subsystem/Subsystem2/UpdateSigAvrgBuf ==
  SigAvrgLocation : Inport
  SigAvrgVal : Inport  Port=2
  Assignment4 : Assignment  IndexMode=Zero-based  IndexOptions=Starting index (port)  Indices=1  OutputSizes=1
  CopyRight2 : Subsystem  Description=|  mask(Copyright Information){none=on}
      | Copyright info block.                                               
      |                                                                     
      | Place copyright information at the top of every subsystem in design.
      mask prompts: none "No parameters"
      mask help: Place copyright information at the top of every subsystem in design.
      mask Display:
      | NxtrConf = 'Nexteer Confidential';
      | 
      | sys = bdroot; %handle for the current model ("system")
      | first = get_param(sys,'Created');
      | first = first(end-3:end);  %year is last four digits
      | 
      | last = get_param(sys,'LastModifiedDate');
      | if isempty(last)
      |     last = datestr(now,'yyyy');
      | else
      |     last = last(end-3:end);
      | end
      | 
      | if strcmp(first,last)
      |     fprintf('%s -- Copyright %s Nexteer',NxtrConf,first)
      | else
      |     fprintf('%s -- %s%s- %s Nexteer',NxtrConf,char(169),first,last)
      | end
  Data Store Read1 : DataStoreRead  DataStoreName=SigAvrgBuf
  Data Store Write2 : DataStoreWrite  DataStoreName=SigAvrgBuf
  wires:
  Data Store Read1/1 -> Assignment4/1
  SigAvrgLocation/1 -> Assignment4/3
  Assignment4/1 -> Data Store Write2/1
  SigAvrgVal/1 -> Assignment4/2

== system ES106A_StHlthSigStc/StHlthSigStc/UpdStHlthStcData/UpdDataSample/For Iterator Subsystem/If Action Subsystem2/CopyRight2 ==

== system ES106A_StHlthSigStc/StHlthSigStc/UpdStHlthStcData/UpdDataSample/For Iterator Subsystem/Subsystem2/CopyRight2 ==
